simulink model "robotarm_A12"  (R2018b)
settings: Solver=FixedStepAuto  StartTime=0.0  StopTime=options.T_train  RelTol=1e-3  AbsTol=1e-6
undefined symbols (not defined in the file or in its folder): options
libraries: neural x132, simulink x2
(part 2 of 6)

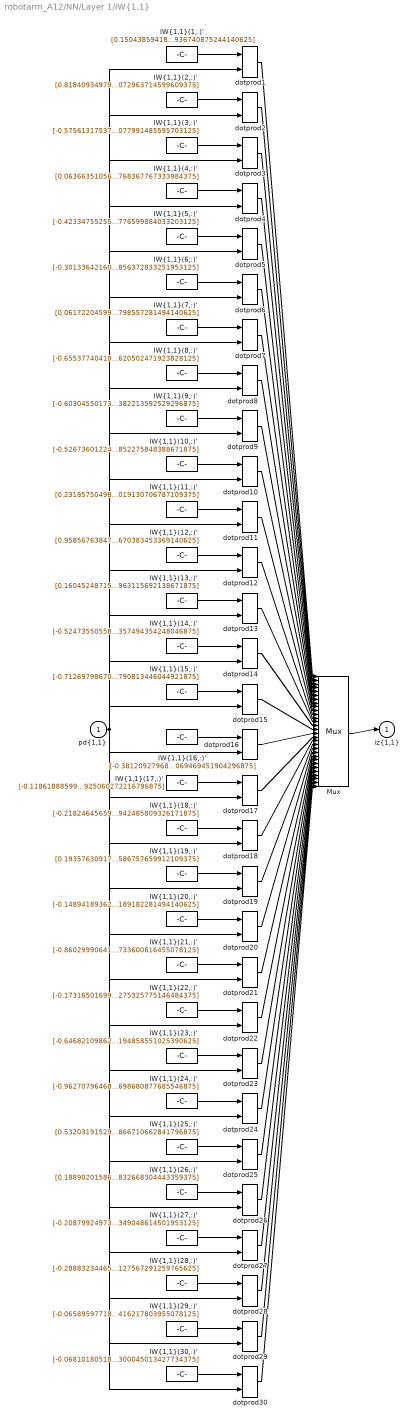
== system robotarm_A12/NN/Layer 1/IW{1,1} ==
  "pd{1,1}" : Inport  PortDimensions=10
      mask Display: e = 0.06;c1 = [120 230 180]/255;c2 = ([120 230 180]+0)/(256+128);c3 = ([120 230 180]+128)/(256+128);patch([0 1 1 0],[0 0 1 1],c1);patch([0 1 1 1-e 1-e 0+e],[0 0 1 1-e 0+e 0+e],c2);patch([0 0 1 1-e 0+e 0+e],[0 1 1 1-e 1-e 0+e],c3);plot([0 1 1 0 0],[0 0 1 1 0]);
  "IW{1,1}(1,:)'" : Constant  Value=[0.1504385941801828774355698215003940276801586151123046875;0.34690561797202723592903339522308669984340667724609375;0.67918699710983287953780518364510498940944671630859375;-0.0631179568047739170122412133423495106399059295654296875;0.342355401745524812184839902329258620738983154296875;0.204072648955312352381241680632228963077068328857421875;-1.1599540167010673474834447915782220661640167236328125;0.31081191949970732313346388764330185949802398681640625;0.306151277821329059758426183179835788905620574951171875;1.0547742812266636125428931336500681936740875244140625]
      mask Display: e = 0.06;c1 = [120 150 230]/255;c2 = ([120 150 230]+0)/383;c3 = ([120 150 230]+128)/383;patch([0 1 1 0],[0 0 1 1],c1);patch([0 1 1 1-e 1-e 0+e],[0 0 1 1-e 0+e 0+e],c2);patch([0 0 1 1-e 0+e 0+e],[0 1 1 1-e 1-e 0+e],c3);plot([0 1 1 0 0],[0 0 1 1 0]);disp('Weights');
  "IW{1,1}(10,:)'" : Constant  Value=[-0.526736012240898165970293121063150465488433837890625;-0.538767346911757538663323430228047072887420654296875;-0.0312499476414010157743206264058244414627552032470703125;-0.2312037357403900761365633798050112091004848480224609375;-0.496427291137826742772887200771947391331195831298828125;0.078308317256865211941629922876018099486827850341796875;0.17728641967244318511376377500710077583789825439453125;-0.9751238259533085983576938815531320869922637939453125;-1.09591360491862133130780421197414398193359375;-0.5796538148699397208218897503684274852275848388671875]
      mask Display: e = 0.06;c1 = [120 150 230]/255;c2 = ([120 150 230]+0)/383;c3 = ([120 150 230]+128)/383;patch([0 1 1 0],[0 0 1 1],c1);patch([0 1 1 1-e 1-e 0+e],[0 0 1 1-e 0+e 0+e],c2);patch([0 0 1 1-e 0+e 0+e],[0 1 1 1-e 1-e 0+e],c3);plot([0 1 1 0 0],[0 0 1 1 0]);disp('Weights');
  "IW{1,1}(11,:)'" : Constant  Value=[0.2318575049853229541607646524425945244729518890380859375;0.217310087618713898560685038319206796586513519287109375;-0.7753798191015601748432573003810830414295196533203125;-0.84528252101619838487778224589419551193714141845703125;-0.66588638266265698373302939216955564916133880615234375;-0.26659650372886278812956106776255182921886444091796875;-0.50415783755661036646955608375719748437404632568359375;0.287402833840340765636511832781252451241016387939453125;0.680723591334707389677305400255136191844940185546875;-0.5084083787759643424664091071463190019130706787109375]
      mask Display: e = 0.06;c1 = [120 150 230]/255;c2 = ([120 150 230]+0)/383;c3 = ([120 150 230]+128)/383;patch([0 1 1 0],[0 0 1 1],c1);patch([0 1 1 1-e 1-e 0+e],[0 0 1 1-e 0+e 0+e],c2);patch([0 0 1 1-e 0+e 0+e],[0 1 1 1-e 1-e 0+e],c3);plot([0 1 1 0 0],[0 0 1 1 0]);disp('Weights');
  "IW{1,1}(12,:)'" : Constant  Value=[0.95856763847245562981669309010612778365612030029296875;-0.08005440626379599355910698932348168455064296722412109375;0.4155709932691113994707166057196445763111114501953125;-0.6586665923285914825413556172861717641353607177734375;-0.52581833699475011290047632428468205034732818603515625;-0.530971279387904449009738527820445597171783447265625;0.283211832425793286205362164764665067195892333984375;-0.31321371948944165541917072914657182991504669189453125;0.73507535982699512278060183234629221260547637939453125;0.59808195780559503251794239986338652670383453369140625]
      mask Display: e = 0.06;c1 = [120 150 230]/255;c2 = ([120 150 230]+0)/383;c3 = ([120 150 230]+128)/383;patch([0 1 1 0],[0 0 1 1],c1);patch([0 1 1 1-e 1-e 0+e],[0 0 1 1-e 0+e 0+e],c2);patch([0 0 1 1-e 0+e 0+e],[0 1 1 1-e 1-e 0+e],c3);plot([0 1 1 0 0],[0 0 1 1 0]);disp('Weights');
  "IW{1,1}(13,:)'" : Constant  Value=[0.160452487153353751114792657972429879009723663330078125;-1.0490247723597854179189425849472172558307647705078125;1.0767381494437200384339803349575959146022796630859375;0.76901878844213322761191875542863272130489349365234375;-0.09502891589200845867679845468956045806407928466796875;-0.0397946913001770707918325342689058743417263031005859375;0.06793225399700318634099716064156382344663143157958984375;0.435259576540429515834063067813985981047153472900390625;0.6752207042976063888772841892205178737640380859375;-0.281466687177426677646252528575132600963115692138671875]
      mask Display: e = 0.06;c1 = [120 150 230]/255;c2 = ([120 150 230]+0)/383;c3 = ([120 150 230]+128)/383;patch([0 1 1 0],[0 0 1 1],c1);patch([0 1 1 1-e 1-e 0+e],[0 0 1 1-e 0+e 0+e],c2);patch([0 0 1 1-e 0+e 0+e],[0 1 1 1-e 1-e 0+e],c3);plot([0 1 1 0 0],[0 0 1 1 0]);disp('Weights');
  "IW{1,1}(14,:)'" : Constant  Value=[-0.5247355055868874185165395829244516789913177490234375;1.08204814787827974242873096955008804798126220703125;-0.070289083751460257332155379117466509342193603515625;-0.134426516773195114939909444728982634842395782470703125;0.43748384555868913281528875813819468021392822265625;-1.115862282969100505169990356080234050750732421875;0.197426980533075224766292876665829680860042572021484375;0.167691152573292701077889432781375944614410400390625;-0.34212858145482549776517089412664063274860382080078125;-0.69630538562402388702565758649143390357494354248046875]
      mask Display: e = 0.06;c1 = [120 150 230]/255;c2 = ([120 150 230]+0)/383;c3 = ([120 150 230]+128)/383;patch([0 1 1 0],[0 0 1 1],c1);patch([0 1 1 1-e 1-e 0+e],[0 0 1 1-e 0+e 0+e],c2);patch([0 0 1 1-e 0+e 0+e],[0 1 1 1-e 1-e 0+e],c3);plot([0 1 1 0 0],[0 0 1 1 0]);disp('Weights');
  "IW{1,1}(15,:)'" : Constant  Value=[-0.71269798670898210080082435524673201143741607666015625;-0.472739992109065421121982808472239412367343902587890625;-0.83277918622136992699012125740409828722476959228515625;-0.414096267133231499268930519974674098193645477294921875;0.443030343191626985177578035290935076773166656494140625;-0.78862022115888585904741603371803648769855499267578125;-0.7006947713982218939321455764002166688442230224609375;-0.51858313807408917828212224776507355272769927978515625;-0.12634287398633337051734315537032671272754669189453125;0.09405443184528898548091291331729735247790813446044921875]
      mask Display: e = 0.06;c1 = [120 150 230]/255;c2 = ([120 150 230]+0)/383;c3 = ([120 150 230]+128)/383;patch([0 1 1 0],[0 0 1 1],c1);patch([0 1 1 1-e 1-e 0+e],[0 0 1 1-e 0+e 0+e],c2);patch([0 0 1 1-e 0+e 0+e],[0 1 1 1-e 1-e 0+e],c3);plot([0 1 1 0 0],[0 0 1 1 0]);disp('Weights');
  "IW{1,1}(16,:)'" : Constant  Value=[-0.381209279683333013277746204039431177079677581787109375;-0.343884104832343495683488754366408102214336395263671875;-0.44863143478299727373581617939635179936885833740234375;-0.9988323246718155967727170718717388808727264404296875;-0.4726826882875005964024239801801741123199462890625;-0.6613034016228713785068293873337097465991973876953125;0.30379769175768955857819264565478079020977020263671875;-0.70754575984422996004497008470934815704822540283203125;-0.7399562091425455623294737961259670555591583251953125;-0.1858576479665747516190066335184383206069469451904296875]
      mask Display: e = 0.06;c1 = [120 150 230]/255;c2 = ([120 150 230]+0)/383;c3 = ([120 150 230]+128)/383;patch([0 1 1 0],[0 0 1 1],c1);patch([0 1 1 1-e 1-e 0+e],[0 0 1 1-e 0+e 0+e],c2);patch([0 0 1 1-e 0+e 0+e],[0 1 1 1-e 1-e 0+e],c3);plot([0 1 1 0 0],[0 0 1 1 0]);disp('Weights');
  "IW{1,1}(17,:)'" : Constant  Value=[-0.11861888599399829369307468596161925233900547027587890625;-0.54130706354673818747613722734968177974224090576171875;0.56498436531732398879768197730300016701221466064453125;0.487658663520003532454438754939474165439605712890625;0.12490103298361114603221011520872707478702068328857421875;-0.01301100060357051994841537378988505224697291851043701171875;1.1313441924976057606500035035423934459686279296875;0.6740406614291172271435925722471438348293304443359375;0.20511085212248392206646485647070221602916717529296875;0.60506745656761740104201408030348829925060272216796875]
      mask Display: e = 0.06;c1 = [120 150 230]/255;c2 = ([120 150 230]+0)/383;c3 = ([120 150 230]+128)/383;patch([0 1 1 0],[0 0 1 1],c1);patch([0 1 1 1-e 1-e 0+e],[0 0 1 1-e 0+e 0+e],c2);patch([0 0 1 1-e 0+e 0+e],[0 1 1 1-e 1-e 0+e],c3);plot([0 1 1 0 0],[0 0 1 1 0]);disp('Weights');
  "IW{1,1}(18,:)'" : Constant  Value=[-0.2182464565988046223399265954867587424814701080322265625;0.57185539987446798448900153744034469127655029296875;-0.52371913472363085251259917640709318220615386962890625;-0.31924064681073371918529346658033318817615509033203125;-0.76297555378147041693637220305390655994415283203125;0.74700125031377540008037385632633231580257415771484375;-0.7616807218947385660356985681573860347270965576171875;0.08389815725791595346638729324695304967463016510009765625;-0.69412157959673559393110053861164487898349761962890625;0.1243127092626363505711850621082703582942485809326171875]
      mask Display: e = 0.06;c1 = [120 150 230]/255;c2 = ([120 150 230]+0)/383;c3 = ([120 150 230]+128)/383;patch([0 1 1 0],[0 0 1 1],c1);patch([0 1 1 1-e 1-e 0+e],[0 0 1 1-e 0+e 0+e],c2);patch([0 0 1 1-e 0+e 0+e],[0 1 1 1-e 1-e 0+e],c3);plot([0 1 1 0 0],[0 0 1 1 0]);disp('Weights');
  "IW{1,1}(19,:)'" : Constant  Value=[0.193576309170048810326392185743316076695919036865234375;0.52779653016123229125611260315054096281528472900390625;-0.763410308871594889268408223870210349559783935546875;0.95781856490806427384399057700647972524166107177734375;0.72610583914309578812407153236563317477703094482421875;0.2259590502889449459278381482363329268991947174072265625;0.17180781900193176081614865324809215962886810302734375;-0.19629772257411548519456800931948237121105194091796875;-0.00184106358578182429351632887204459620988927781581878662109375;0.804246066341609999739148406661115586757659912109375]
      mask Display: e = 0.06;c1 = [120 150 230]/255;c2 = ([120 150 230]+0)/383;c3 = ([120 150 230]+128)/383;patch([0 1 1 0],[0 0 1 1],c1);patch([0 1 1 1-e 1-e 0+e],[0 0 1 1-e 0+e 0+e],c2);patch([0 0 1 1-e 0+e 0+e],[0 1 1 1-e 1-e 0+e],c3);plot([0 1 1 0 0],[0 0 1 1 0]);disp('Weights');
  "IW{1,1}(2,:)'" : Constant  Value=[0.8184093497975035713665192815824411809444427490234375;-0.7050103667468905488391328617581166326999664306640625;0.53729700090761500774760861531831324100494384765625;-0.491297922694489297423814377907547168433666229248046875;0.59433539373797750204886369829182513058185577392578125;-0.003407527349241196330809078318679894437082111835479736328125;-0.62496813755304281290392509617959149181842803955078125;-0.1463999438678708353567259337069117464125156402587890625;0.9159542187835014726005056218127720057964324951171875;-0.6815425789896263353284666663967072963714599609375]
      mask Display: e = 0.06;c1 = [120 150 230]/255;c2 = ([120 150 230]+0)/383;c3 = ([120 150 230]+128)/383;patch([0 1 1 0],[0 0 1 1],c1);patch([0 1 1 1-e 1-e 0+e],[0 0 1 1-e 0+e 0+e],c2);patch([0 0 1 1-e 0+e 0+e],[0 1 1 1-e 1-e 0+e],c3);plot([0 1 1 0 0],[0 0 1 1 0]);disp('Weights');
  "IW{1,1}(20,:)'" : Constant  Value=[-0.1489418936258715131515373286674730479717254638671875;0.447943488132920897282218675172771327197551727294921875;-1.1909633692501395696439203675254248082637786865234375;0.339902391431985584357988727788324467837810516357421875;-0.044406298375034847225606426945887506008148193359375;0.85903606858458891881724639461026526987552642822265625;0.43436217229584939136799448533565737307071685791015625;-0.490751586325180400027790028616436757147312164306640625;0.56333456222314126637940034925122745335102081298828125;0.0153348805316285453914648684303756454028189182281494140625]
      mask Display: e = 0.06;c1 = [120 150 230]/255;c2 = ([120 150 230]+0)/383;c3 = ([120 150 230]+128)/383;patch([0 1 1 0],[0 0 1 1],c1);patch([0 1 1 1-e 1-e 0+e],[0 0 1 1-e 0+e 0+e],c2);patch([0 0 1 1-e 0+e 0+e],[0 1 1 1-e 1-e 0+e],c3);plot([0 1 1 0 0],[0 0 1 1 0]);disp('Weights');
  "IW{1,1}(21,:)'" : Constant  Value=[-0.86029990641294495912205775312031619250774383544921875;0.33489519141073509356232307254686020314693450927734375;-0.40242452183544852317709228373132646083831787109375;0.234168530862867096953294776540133170783519744873046875;-0.41215311936807730308629516002838499844074249267578125;-0.84951487856116203456480207023560069501399993896484375;0.89519767909989533816172979641123674809932708740234375;-0.164117402233892206719900741518358699977397918701171875;-0.37370730782799199687360669486224651336669921875;-0.51236459217931262788425783583079464733600616455078125]
      mask Display: e = 0.06;c1 = [120 150 230]/255;c2 = ([120 150 230]+0)/383;c3 = ([120 150 230]+128)/383;patch([0 1 1 0],[0 0 1 1],c1);patch([0 1 1 1-e 1-e 0+e],[0 0 1 1-e 0+e 0+e],c2);patch([0 0 1 1-e 0+e 0+e],[0 1 1 1-e 1-e 0+e],c3);plot([0 1 1 0 0],[0 0 1 1 0]);disp('Weights');
  "IW{1,1}(22,:)'" : Constant  Value=[-0.1731650169979390418983911104078288190066814422607421875;-0.1432341277504907417483792642087792046368122100830078125;-0.811964056111784682201459872885607182979583740234375;1.0296200371538126727699591356213204562664031982421875;0.53795992638017786635629136071656830608844757080078125;-0.7871197196842156795781875189277343451976776123046875;-0.1632683707133474049211230294531560502946376800537109375;0.0744792588242456921054923668634728528559207916259765625;-0.452405288008265349386505249640322290360927581787109375;-1.0788759896658335346586454761563800275325775146484375]
      mask Display: e = 0.06;c1 = [120 150 230]/255;c2 = ([120 150 230]+0)/383;c3 = ([120 150 230]+128)/383;patch([0 1 1 0],[0 0 1 1],c1);patch([0 1 1 1-e 1-e 0+e],[0 0 1 1-e 0+e 0+e],c2);patch([0 0 1 1-e 0+e 0+e],[0 1 1 1-e 1-e 0+e],c3);plot([0 1 1 0 0],[0 0 1 1 0]);disp('Weights');
  "IW{1,1}(23,:)'" : Constant  Value=[-0.64682109862249104192954973768792115151882171630859375;0.079710802145811776586725727611337788403034210205078125;0.6820724783123630619030564048443920910358428955078125;-0.1818835116594154921454418172288569621741771697998046875;-0.7665735226401100277371369884349405765533447265625;0.92632406015705470725407622012426145374774932861328125;-0.43514151694210811971430530320503748953342437744140625;-0.73247173377981733555230903220945037901401519775390625;-0.0201690636992467968446884896138726617209613323211669921875;-0.87286810026704098053329516915255226194858551025390625]
      mask Display: e = 0.06;c1 = [120 150 230]/255;c2 = ([120 150 230]+0)/383;c3 = ([120 150 230]+128)/383;patch([0 1 1 0],[0 0 1 1],c1);patch([0 1 1 1-e 1-e 0+e],[0 0 1 1-e 0+e 0+e],c2);patch([0 0 1 1-e 0+e 0+e],[0 1 1 1-e 1-e 0+e],c3);plot([0 1 1 0 0],[0 0 1 1 0]);disp('Weights');
  "IW{1,1}(24,:)'" : Constant  Value=[-0.9627079646801093293362328040529973804950714111328125;-0.6232131356180958814405812518089078366756439208984375;-0.6813727271358225312525291883503086864948272705078125;0.7914260933280086174335110626998357474803924560546875;-0.1721487876975571762461214575523626990616321563720703125;-0.2217771926539286175827925262638018466532230377197265625;0.263401924387009156447447821847163140773773193359375;-0.1713679047494627571968095480769989080727100372314453125;-0.88897037224212349659779874855303205549716949462890625;0.330298177955564209451466695099952630698680877685546875]
      mask Display: e = 0.06;c1 = [120 150 230]/255;c2 = ([120 150 230]+0)/383;c3 = ([120 150 230]+128)/383;patch([0 1 1 0],[0 0 1 1],c1);patch([0 1 1 1-e 1-e 0+e],[0 0 1 1-e 0+e 0+e],c2);patch([0 0 1 1-e 0+e 0+e],[0 1 1 1-e 1-e 0+e],c3);plot([0 1 1 0 0],[0 0 1 1 0]);disp('Weights');
  "IW{1,1}(25,:)'" : Constant  Value=[0.5320319152999231082645792412222363054752349853515625;-0.1402630533875996732273705447369138710200786590576171875;0.36849458240897503547017777236760593950748443603515625;-0.625071299177949679659604953485541045665740966796875;0.709631863734205836635737796314060688018798828125;-0.7996691699953004661693967136670835316181182861328125;0.3453214499362109446423119152314029633998870849609375;0.5166656851930537808215149198076687753200531005859375;0.40610077013694334535642838091007433831691741943359375;-0.455506780890050588794792929547838866710662841796875]
      mask Display: e = 0.06;c1 = [120 150 230]/255;c2 = ([120 150 230]+0)/383;c3 = ([120 150 230]+128)/383;patch([0 1 1 0],[0 0 1 1],c1);patch([0 1 1 1-e 1-e 0+e],[0 0 1 1-e 0+e 0+e],c2);patch([0 0 1 1-e 0+e 0+e],[0 1 1 1-e 1-e 0+e],c3);plot([0 1 1 0 0],[0 0 1 1 0]);disp('Weights');
  "IW{1,1}(26,:)'" : Constant  Value=[0.1889020158605952126595894924321328289806842803955078125;0.558902656368921224583345974679104983806610107421875;-0.07796490092741904798234742202112101949751377105712890625;0.2180543350093030741110311510055908001959323883056640625;0.1532993487623071360292925646717776544392108917236328125;-0.78152413386430541475391464700805954635143280029296875;0.19996211043138345520020493495394475758075714111328125;-0.56417618719033069130119883993756957352161407470703125;1.0676594735490583243375795063911937177181243896484375;-0.73013723606074021343914637327543459832668304443359375]
      mask Display: e = 0.06;c1 = [120 150 230]/255;c2 = ([120 150 230]+0)/383;c3 = ([120 150 230]+128)/383;patch([0 1 1 0],[0 0 1 1],c1);patch([0 1 1 1-e 1-e 0+e],[0 0 1 1-e 0+e 0+e],c2);patch([0 0 1 1-e 0+e 0+e],[0 1 1 1-e 1-e 0+e],c3);plot([0 1 1 0 0],[0 0 1 1 0]);disp('Weights');
  "IW{1,1}(27,:)'" : Constant  Value=[-0.20879924973470831428556948594632558524608612060546875;0.6135492101841040213372480138787068426609039306640625;-1.037790763115799652638315819785930216312408447265625;-0.62377881746567831466876441481872461736202239990234375;-0.09821930441919217436019806655167485587298870086669921875;1.049940392269574029882051036111079156398773193359375;-0.61627881563772712869564429638558067381381988525390625;-0.74995449440609995850337554657016880810260772705078125;-0.34419011151639111734112930207629688084125518798828125;-0.28418786373834425962314753633108921349048614501953125]
      mask Display: e = 0.06;c1 = [120 150 230]/255;c2 = ([120 150 230]+0)/383;c3 = ([120 150 230]+128)/383;patch([0 1 1 0],[0 0 1 1],c1);patch([0 1 1 1-e 1-e 0+e],[0 0 1 1-e 0+e 0+e],c2);patch([0 0 1 1-e 0+e 0+e],[0 1 1 1-e 1-e 0+e],c3);plot([0 1 1 0 0],[0 0 1 1 0]);disp('Weights');
  "IW{1,1}(28,:)'" : Constant  Value=[-0.288832344651085259901179824737482704222202301025390625;-1.206039119363871758849882098729722201824188232421875;-0.26174547419834259809334753299481235444545745849609375;0.38437709292274024885927019568043760955333709716796875;0.55002547818475899799040007565054111182689666748046875;0.263374727852550005735565719078294932842254638671875;-0.37229294746976637764390716256457380950450897216796875;0.10906463115023599941277865355004905723035335540771484375;-0.8665615525072178915166887236409820616245269775390625;-0.10407129854531883828006044723224476911127567291259765625]
      mask Display: e = 0.06;c1 = [120 150 230]/255;c2 = ([120 150 230]+0)/383;c3 = ([120 150 230]+128)/383;patch([0 1 1 0],[0 0 1 1],c1);patch([0 1 1 1-e 1-e 0+e],[0 0 1 1-e 0+e 0+e],c2);patch([0 0 1 1-e 0+e 0+e],[0 1 1 1-e 1-e 0+e],c3);plot([0 1 1 0 0],[0 0 1 1 0]);disp('Weights');
  "IW{1,1}(29,:)'" : Constant  Value=[-0.0658959771819299378048384596695541404187679290771484375;0.371584699319927047600486957890097983181476593017578125;0.497324952386737184628628938298788852989673614501953125;0.38358392431787458054515127514605410397052764892578125;-0.7506563997345330196964141578064300119876861572265625;0.5866313997971699389921695910743437707424163818359375;-0.70920590994006482699063553809537552297115325927734375;-0.440466933750873812503101589754805900156497955322265625;0.680973208770148108470721126650460064411163330078125;-0.80468529348088957409146360078011639416217803955078125]
      mask Display: e = 0.06;c1 = [120 150 230]/255;c2 = ([120 150 230]+0)/383;c3 = ([120 150 230]+128)/383;patch([0 1 1 0],[0 0 1 1],c1);patch([0 1 1 1-e 1-e 0+e],[0 0 1 1-e 0+e 0+e],c2);patch([0 0 1 1-e 0+e 0+e],[0 1 1 1-e 1-e 0+e],c3);plot([0 1 1 0 0],[0 0 1 1 0]);disp('Weights');
  "IW{1,1}(3,:)'" : Constant  Value=[-0.5756131753768636283297155387117527425289154052734375;0.7103689353132691675085652605048380792140960693359375;-0.6886265036195495792270548918168060481548309326171875;0.416424844698797425035508013024809770286083221435546875;0.67681853912544609475077095339656807482242584228515625;0.297074587374453191745971025738981552422046661376953125;0.65984346358257806031133441138081252574920654296875;-0.64000938767664983242156040432746522128582000732421875;0.8723099656412642843861249275505542755126953125;0.31411972271197630135475264978595077991485595703125]
      mask Display: e = 0.06;c1 = [120 150 230]/255;c2 = ([120 150 230]+0)/383;c3 = ([120 150 230]+128)/383;patch([0 1 1 0],[0 0 1 1],c1);patch([0 1 1 1-e 1-e 0+e],[0 0 1 1-e 0+e 0+e],c2);patch([0 0 1 1-e 0+e 0+e],[0 1 1 1-e 1-e 0+e],c3);plot([0 1 1 0 0],[0 0 1 1 0]);disp('Weights');
  "IW{1,1}(30,:)'" : Constant  Value=[-0.06810180518166554508585619487348594702780246734619140625;0.07735983131844410831678970907887560315430164337158203125;-0.54790916424342561708016319244052283465862274169921875;-0.2257957729935486657080190298074739985167980194091796875;-0.98637338512081262908992584925726987421512603759765625;-0.66861865699239431126699173546512611210346221923828125;0.476967756441096291109005278485710732638835906982421875;0.76157937133137620921985444510937668383121490478515625;0.1383326289680176512941756072905263863503932952880859375;-0.73521137188302299048103805034770630300045013427734375]
      mask Display: e = 0.06;c1 = [120 150 230]/255;c2 = ([120 150 230]+0)/383;c3 = ([120 150 230]+128)/383;patch([0 1 1 0],[0 0 1 1],c1);patch([0 1 1 1-e 1-e 0+e],[0 0 1 1-e 0+e 0+e],c2);patch([0 0 1 1-e 0+e 0+e],[0 1 1 1-e 1-e 0+e],c3);plot([0 1 1 0 0],[0 0 1 1 0]);disp('Weights');
  "IW{1,1}(4,:)'" : Constant  Value=[0.06366351056725859380858167924088775180280208587646484375;-0.91159558242380434034402014731313101947307586669921875;-0.341386876413746875869037467055022716522216796875;0.835741400674049117469621705822646617889404296875;0.11183180113611761175018699532301980070769786834716796875;0.7023307623763013207707217588904313743114471435546875;-0.66256727729853304165175131856813095510005950927734375;0.2201715179391760257576748927021981216967105865478515625;-0.8393654199243680835706982179544866085052490234375;0.68845295272500750538569036507396958768367767333984375]
      mask Display: e = 0.06;c1 = [120 150 230]/255;c2 = ([120 150 230]+0)/383;c3 = ([120 150 230]+128)/383;patch([0 1 1 0],[0 0 1 1],c1);patch([0 1 1 1-e 1-e 0+e],[0 0 1 1-e 0+e 0+e],c2);patch([0 0 1 1-e 0+e 0+e],[0 1 1 1-e 1-e 0+e],c3);plot([0 1 1 0 0],[0 0 1 1 0]);disp('Weights');
  "IW{1,1}(5,:)'" : Constant  Value=[-0.42334755255171307997130725198076106607913970947265625;0.21161823179134930938971592695452272891998291015625;0.295981854036569680399537674020393751561641693115234375;0.5505463955379192864114656913443468511104583740234375;-0.87292404867895634357211065434967167675495147705078125;-0.82263204347566165619554112709010951220989227294921875;0.1652087016923362294829047414168599061667919158935546875;-0.26899337995137917456389686776674352586269378662109375;0.2637348725173234154084411784424446523189544677734375;0.542708180907578441320993078988976776599884033203125]
      mask Display: e = 0.06;c1 = [120 150 230]/255;c2 = ([120 150 230]+0)/383;c3 = ([120 150 230]+128)/383;patch([0 1 1 0],[0 0 1 1],c1);patch([0 1 1 1-e 1-e 0+e],[0 0 1 1-e 0+e 0+e],c2);patch([0 0 1 1-e 0+e 0+e],[0 1 1 1-e 1-e 0+e],c3);plot([0 1 1 0 0],[0 0 1 1 0]);disp('Weights');
  "IW{1,1}(6,:)'" : Constant  Value=[-0.301336421600733483927569977822713553905487060546875;0.1721468321240211818423659906329703517258167266845703125;-0.77643166545570718728441761413705535233020782470703125;-0.7250544705510770793210895135416649281978607177734375;-0.0760292042581368343601155856958939693868160247802734375;0.1391708369597551564478266072910628281533718109130859375;-0.2660565840408597448885075209545902907848358154296875;0.75237493918520870206378958755522035062313079833984375;-0.9652024319148855280303678227937780320644378662109375;0.1047776742134469973866117697980371303856372833251953125]
      mask Display: e = 0.06;c1 = [120 150 230]/255;c2 = ([120 150 230]+0)/383;c3 = ([120 150 230]+128)/383;patch([0 1 1 0],[0 0 1 1],c1);patch([0 1 1 1-e 1-e 0+e],[0 0 1 1-e 0+e 0+e],c2);patch([0 0 1 1-e 0+e 0+e],[0 1 1 1-e 1-e 0+e],c3);plot([0 1 1 0 0],[0 0 1 1 0]);disp('Weights');
  "IW{1,1}(7,:)'" : Constant  Value=[0.061722045993229966709403555569224408827722072601318359375;0.0281573701027865060109167671953400713391602039337158203125;-0.0210567715210280559379185660873190499842166900634765625;-0.9101081414598060081999619796988554298877716064453125;0.258677727228922071933681081645772792398929595947265625;-0.65765918959270219801283019478432834148406982421875;-0.75835294405146991270072476254426874220371246337890625;-0.3095338838869514663798554465756751596927642822265625;0.6663547818853226001323264426901005208492279052734375;0.718551416048244906420450206496752798557281494140625]
      mask Display: e = 0.06;c1 = [120 150 230]/255;c2 = ([120 150 230]+0)/383;c3 = ([120 150 230]+128)/383;patch([0 1 1 0],[0 0 1 1],c1);patch([0 1 1 1-e 1-e 0+e],[0 0 1 1-e 0+e 0+e],c2);patch([0 0 1 1-e 0+e 0+e],[0 1 1 1-e 1-e 0+e],c3);plot([0 1 1 0 0],[0 0 1 1 0]);disp('Weights');
  "IW{1,1}(8,:)'" : Constant  Value=[-0.6553774041898263735816954067558981478214263916015625;-0.532143911385816181791597045958042144775390625;0.55113663050991290592861560071469284594058990478515625;0.528029413236786648866427640314213931560516357421875;-0.721728560275065600393418208113871514797210693359375;0.86695381001518712071884920078446157276630401611328125;0.363128914675880931639539994648657739162445068359375;-0.565613833401616528107069825637154281139373779296875;0.51016566842844734974704579144599847495555877685546875;-0.266743623867181256503755548692424781620502471923828125]
      mask Display: e = 0.06;c1 = [120 150 230]/255;c2 = ([120 150 230]+0)/383;c3 = ([120 150 230]+128)/383;patch([0 1 1 0],[0 0 1 1],c1);patch([0 1 1 1-e 1-e 0+e],[0 0 1 1-e 0+e 0+e],c2);patch([0 0 1 1-e 0+e 0+e],[0 1 1 1-e 1-e 0+e],c3);plot([0 1 1 0 0],[0 0 1 1 0]);disp('Weights');
  "IW{1,1}(9,:)'" : Constant  Value=[-0.60304550173630999676532837838749401271343231201171875;-0.2900759958473135835532730197883211076259613037109375;0.90202639005731655164055382556398399174213409423828125;-0.1192427447763907688571549670086824335157871246337890625;0.8654811432514935010118506397702731192111968994140625;-0.68720743023600350252166890641092322766780853271484375;-0.564447786907311677140341998892836272716522216796875;0.55271860765459990272319146242807619273662567138671875;0.646881590401628070452488827868364751338958740234375;0.59140880743816726106132364293443970382213592529296875]
      mask Display: e = 0.06;c1 = [120 150 230]/255;c2 = ([120 150 230]+0)/383;c3 = ([120 150 230]+128)/383;patch([0 1 1 0],[0 0 1 1],c1);patch([0 1 1 1-e 1-e 0+e],[0 0 1 1-e 0+e 0+e],c2);patch([0 0 1 1-e 0+e 0+e],[0 1 1 1-e 1-e 0+e],c3);plot([0 1 1 0 0],[0 0 1 1 0]);disp('Weights');
  Mux : Mux  Inputs=30
      mask Display: e = 0.06;c1 = [120 150 230]/255;c2 = ([120 150 230]+0)/383;c3 = ([120 150 230]+128)/383;patch([0 1 1 0],[0 0 1 1],c1);patch([0 1 1 1-e 1-e 0+e],[0 0 1 1-e 0+e 0+e],c2);patch([0 0 1 1-e 0+e 0+e],[0 1 1 1-e 1-e 0+e],c3);plot([0 1 1 0 0],[0 0 1 1 0]);disp('Mux');
  dotprod{1..30} (30 alike) : neural/Weight Functions/dotprod
  "iz{1,1}" : Outport
      mask Display: e = 0.06;c1 = [120 230 180]/255;c2 = ([120 230 180]+0)/(256+128);c3 = ([120 230 180]+128)/(256+128);patch([0 1 1 0],[0 0 1 1],c1);patch([0 1 1 1-e 1-e 0+e],[0 0 1 1-e 0+e 0+e],c2);patch([0 0 1 1-e 0+e 0+e],[0 1 1 1-e 1-e 0+e],c3);plot([0 1 1 0 0],[0 0 1 1 0]);
  wires:
  "IW{1,1}(1,:)'"/1 -> dotprod1/1
  "pd{1,1}"/1 -> dotprod1/2, dotprod2/2, dotprod3/2, dotprod4/2, dotprod5/2, dotprod6/2, dotprod7/2, dotprod8/2, dotprod9/2, dotprod10/2, dotprod11/2, dotprod12/2, dotprod13/2, dotprod14/2, dotprod15/2, dotprod16/2, dotprod17/2, dotprod18/2, dotprod19/2, dotprod20/2, dotprod21/2, dotprod22/2, dotprod23/2, dotprod24/2, dotprod25/2, dotprod26/2, dotprod27/2, dotprod28/2, dotprod29/2, dotprod30/2
  dotprod1/1 -> Mux/1
  "IW{1,1}(2,:)'"/1 -> dotprod2/1
  dotprod2/1 -> Mux/2
  "IW{1,1}(3,:)'"/1 -> dotprod3/1
  dotprod3/1 -> Mux/3
  "IW{1,1}(4,:)'"/1 -> dotprod4/1
  dotprod4/1 -> Mux/4
  "IW{1,1}(5,:)'"/1 -> dotprod5/1
  dotprod5/1 -> Mux/5
  "IW{1,1}(6,:)'"/1 -> dotprod6/1
  dotprod6/1 -> Mux/6
  "IW{1,1}(7,:)'"/1 -> dotprod7/1
  dotprod7/1 -> Mux/7
  "IW{1,1}(8,:)'"/1 -> dotprod8/1
  dotprod8/1 -> Mux/8
  "IW{1,1}(9,:)'"/1 -> dotprod9/1
  dotprod9/1 -> Mux/9
  "IW{1,1}(10,:)'"/1 -> dotprod10/1
  dotprod10/1 -> Mux/10
  "IW{1,1}(11,:)'"/1 -> dotprod11/1
  dotprod11/1 -> Mux/11
  "IW{1,1}(12,:)'"/1 -> dotprod12/1
  dotprod12/1 -> Mux/12
  "IW{1,1}(13,:)'"/1 -> dotprod13/1
  dotprod13/1 -> Mux/13
  "IW{1,1}(14,:)'"/1 -> dotprod14/1
  dotprod14/1 -> Mux/14
  "IW{1,1}(15,:)'"/1 -> dotprod15/1
  dotprod15/1 -> Mux/15
  "IW{1,1}(16,:)'"/1 -> dotprod16/1
  dotprod16/1 -> Mux/16
  "IW{1,1}(17,:)'"/1 -> dotprod17/1
  dotprod17/1 -> Mux/17
  "IW{1,1}(18,:)'"/1 -> dotprod18/1
  dotprod18/1 -> Mux/18
  "IW{1,1}(19,:)'"/1 -> dotprod19/1
  dotprod19/1 -> Mux/19
  "IW{1,1}(20,:)'"/1 -> dotprod20/1
  dotprod20/1 -> Mux/20
  "IW{1,1}(21,:)'"/1 -> dotprod21/1
  dotprod21/1 -> Mux/21
  "IW{1,1}(22,:)'"/1 -> dotprod22/1
  dotprod22/1 -> Mux/22
  "IW{1,1}(23,:)'"/1 -> dotprod23/1
  dotprod23/1 -> Mux/23
  "IW{1,1}(24,:)'"/1 -> dotprod24/1
  dotprod24/1 -> Mux/24
  "IW{1,1}(25,:)'"/1 -> dotprod25/1
  dotprod25/1 -> Mux/25
  "IW{1,1}(26,:)'"/1 -> dotprod26/1
  dotprod26/1 -> Mux/26
  "IW{1,1}(27,:)'"/1 -> dotprod27/1
  dotprod27/1 -> Mux/27
  "IW{1,1}(28,:)'"/1 -> dotprod28/1
  dotprod28/1 -> Mux/28
  "IW{1,1}(29,:)'"/1 -> dotprod29/1
  dotprod29/1 -> Mux/29
  "IW{1,1}(30,:)'"/1 -> dotprod30/1
  dotprod30/1 -> Mux/30
  Mux/1 -> "iz{1,1}"/1

== system robotarm_A12/NN/Layer 2/Delays 1 ==
  "p{2}" : Inport  PortDimensions=30
      mask Display: e = 0.06;c1 = [120 230 180]/255;c2 = ([120 230 180]+0)/(256+128);c3 = ([120 230 180]+128)/(256+128);patch([0 1 1 0],[0 0 1 1],c1);patch([0 1 1 1-e 1-e 0+e],[0 0 1 1-e 0+e 0+e],c2);patch([0 0 1 1-e 0+e 0+e],[0 1 1 1-e 1-e 0+e],c3);plot([0 1 1 0 0],[0 0 1 1 0]);
  mux : Mux  Inputs=1
      mask Display: e = 0.06;c1 = [120 150 230]/255;c2 = ([120 150 230]+0)/383;c3 = ([120 150 230]+128)/383;patch([0 1 1 0],[0 0 1 1],c1);patch([0 1 1 1-e 1-e 0+e],[0 0 1 1-e 0+e 0+e],c2);patch([0 0 1 1-e 0+e 0+e],[0 1 1 1-e 1-e 0+e],c3);plot([0 1 1 0 0],[0 0 1 1 0]);disp('Mux')
  "pd{2,1}" : Outport
      mask Display: e = 0.06;c1 = [120 230 180]/255;c2 = ([120 230 180]+0)/(256+128);c3 = ([120 230 180]+128)/(256+128);patch([0 1 1 0],[0 0 1 1],c1);patch([0 1 1 1-e 1-e 0+e],[0 0 1 1-e 0+e 0+e],c2);patch([0 0 1 1-e 0+e 0+e],[0 1 1 1-e 1-e 0+e],c3);plot([0 1 1 0 0],[0 0 1 1 0]);
  wires:
  "p{2}"/1 -> mux/1
  mux/1 -> "pd{2,1}"/1
